simulink model "uni_driveline_gui"  (R2019a)
settings: Solver=ode45  StartTime=0.0  StopTime=sim_time  RelTol=1e-3
InitFcn:
  | if ~exist('x0')
  |   x0 = [5 5 0];
  |   msgbox(sprintf('x0 not defined in workspace, setting it to [%g %g %g]\n', x0));
  | end
  | if ~exist('L')
  |   L = [1 -2 4];
  |   msgbox(sprintf('L not defined in workspace, setting it to [%g %g %g]\n', L));
  | end
  | % clean up old vehicle icons
  | set(0, 'ShowHiddenHandles', 'on')
  | delete(findobj('Tag', 'vehicle'))
  | set(0, 'ShowHiddenHandles', 'off')
StopFcn:
  | % update the XY scope
  | set(0, 'ShowHiddenHandles', 'on')
  | fig = findobj('name', 'XY');
  | ax = findobj(fig, 'type', 'axes');
  | axes(ax)
  | grid on
  | hold on
  | plot_vehicle(x0, 'g', 'Tag', 'vehicle')
  | plot_homline(L, 'r--', 'Tag', 'vehicle')
  | hold off
  | set(0, 'ShowHiddenHandles', 'off')
libraries: simulink x1
settings Model: Creator=Bhuvanashree  LastModifiedBy=Bhuvanashree
settings DataIOCC: SaveFormat=Array  ReturnWorkspaceOutputs=off
settings DebuggingCC: SolverPrmCheckMsg=warning  StateNameClashWarn=warning  SFUnexpectedBacktrackingDiag=warning  SFNoUnconditionalDefaultTransitionDiag=warning  SFExecutionAtInitializationDiag=none
settings ModelReferenceCC: PropagateSignalLabelsOutOfModel=off
settings CodeAppCC: StateflowObjectComments=on

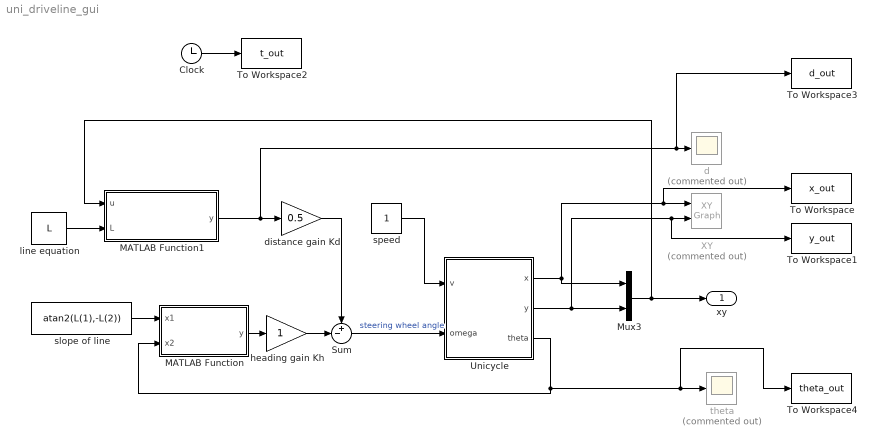
== system uni_driveline_gui ==
  Clock : Clock
  MATLAB Function : MATLAB Function  TreatAsAtomicUnit=on
  MATLAB Function1 : MATLAB Function  TreatAsAtomicUnit=on
  Mux3 : Mux  Inputs=2
  Sum : Sum  Inputs=+-|
  To Workspace : ToWorkspace  VariableName=x_out  SampleTime=-1
  To Workspace1 : ToWorkspace  VariableName=y_out  SampleTime=-1
  To Workspace2 : ToWorkspace  VariableName=t_out  SampleTime=-1
  To Workspace3 : ToWorkspace  VariableName=d_out  SampleTime=-1
  To Workspace4 : ToWorkspace  VariableName=theta_out  SampleTime=-1
  Unicycle : Subsystem  mask{vlim=1, alim=1, x0=x0, wlim=Inf}
      mask prompts: vlim "Velocity limit (m/s)"; alim "Acceleration limit"; x0 "Initial state (x,y,theta)"; wlim "Steering angle limit"
      mask Display:
      | port_label('input', 1, 'v')
      | port_label('input', 2, '\omega', 'texmode', 'on')
      | port_label('output', 1, 'x')
      | port_label('output', 2, 'y')
      | port_label('output', 3, '\theta', 'texmode', 'on')
  XY : simulink/Sinks/XY Graph  Commented=on  xmin=-10  xmax=10  ymin=-10  ymax=10  st=-1
  d : Scope  Commented=on
  distance gain Kd : Gain  Gain=0.5
  heading gain Kh : Gain
  line equation : Constant  Value=L
  slope of line : Constant  Value=atan2(L(1),-L(2))
  speed : Constant  VectorParams1D=off  SampleTime=0.02
  theta : Scope  Commented=on
  xy : Outport
  wires:
  MATLAB Function1/1(y) -> To Workspace3/1, d/1, distance gain Kd/1
  slope of line/1 -> MATLAB Function/1(x1)
  MATLAB Function/1(y) -> heading gain Kh/1
  heading gain Kh/1 -> Sum/2
  Unicycle/1(x) -> Mux3/1, To Workspace/1, XY/1
  distance gain Kd/1 -> Sum/1
  Sum/1 -> Unicycle/2(omega)  "steering wheel angle"
  speed/1 -> Unicycle/1(v)
  Unicycle/3(theta) -> MATLAB Function/2(x2), To Workspace4/1, theta/1
  Unicycle/2(y) -> To Workspace1/1, XY/2, Mux3/2
  Mux3/1 -> MATLAB Function1/1(u), xy/1
  line equation/1 -> MATLAB Function1/2(L)
  Clock/1 -> To Workspace2/1

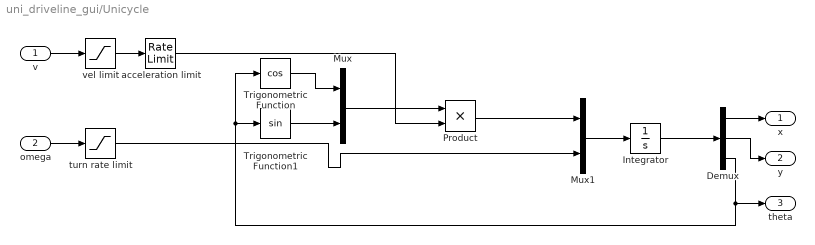
== system uni_driveline_gui/Unicycle ==
  v : Inport
  omega : Inport  Port=2
  Demux : Demux  Outputs=3
  Integrator : Integrator  InitialCondition=x0
  Mux : Mux  Inputs=2
  Mux1 : Mux  Inputs=2
  Product : Product  RndMeth=Zero
  Trigonometric Function : Trigonometry  Operator=cos
  Trigonometric Function1 : Trigonometry
  acceleration limit : RateLimiter  RisingSlewLimit=alim  FallingSlewLimit=-alim  SampleTimeMode=inherited
  turn rate limit : Saturate  UpperLimit=wlim  LowerLimit=-wlim
  vel limit : Saturate  UpperLimit=vlim  LowerLimit=-vlim
  x : Outport
  y : Outport  Port=2
  theta : Outport  Port=3
  wires:
  turn rate limit/1 -> Mux1/2
  Demux/3 -> theta/1, Trigonometric Function1/1, Trigonometric Function/1
  Trigonometric Function/1 -> Mux/1
  Integrator/1 -> Demux/1
  Product/1 -> Mux1/1
  acceleration limit/1 -> Product/2
  v/1 -> vel limit/1
  omega/1 -> turn rate limit/1
  Trigonometric Function1/1 -> Mux/2
  Mux/1 -> Product/1
  Demux/1 -> x/1
  Demux/2 -> y/1
  vel limit/1 -> acceleration limit/1
  Mux1/1 -> Integrator/1

== matlab function uni_driveline_gui/MATLAB Function1 ==
  data: u input; y output; L input
function y = dist_from_line(u,L)
y = (u(1)*L(1)+u(2)*L(2)+L(3))/sqrt(L(1)^2+L(2)^2);

== matlab function uni_driveline_gui/MATLAB Function ==
  data: x1 input; y output; x2 input
function y = ang_diff(x1,x2)

y = angdiff(x1,x2);
